simulink model "Comprobar_Posicion_PID_ISA"  (R2021b)
settings: Solver=ode45  StartTime=0.0  StopTime=100  RelTol=1e-3  EnableMultiTasking=on
undefined symbols (not defined in the file or in its folder): airspeed_0, alpha_0, altitude_0, beta_0, deflect_sat, Earth, euler_0, h0, JSBSim, local_V_0, mTotal, Pos_0, pqr_0, r_MotorLeft, r_MotorRight, theta_0, Vel_0, VTOL_FW, WGS84
libraries: simulink_need_slupdate x5, aerolibfltsims x4, sharedutil x3, sharedtransform x2, aerolibtransform2 x1, aerolibutil x1
(part 2 of 2)

== matlab function Comprobar_Posicion_PID_ISA/Control de Actitud/Dynamic Model/VSkye/Ecuaciones_de_Navegacion1 ==
  data: Mm output; input input
function Mm=par_Motor(input)
%g=9.81;
C_P=0.04;
C_T=0.08;
INCH2M=2.54e-2;
D=8*INCH2M;
Kpar=-D*C_P/(2*pi()*C_T);
%Ft=(1/3.27193530612245)*(-0.0292*(input*100).^2 + 36.681*(input*100) - 107.5)*g/1000;%en N;
Ft=-9.8*input;
Par=Kpar*Ft;%en Nm;

Mm=[0;0;Par];
end

== matlab function Comprobar_Posicion_PID_ISA/Control de Actitud/Lamda controller/PID ISA1/PID CPOH ==
  data: sp input; vm output; vc input; Kc input; Ti input; Td input; Ts input; u0 input; Min_U input; Max_U input; ui1 input; ekf1 input; ui output; ekf output
function [vm,ui,ekf] = fcn(sp,vc,Kc,Ti,Td,Ts,u0,Min_U,Max_U,ui1,ekf1)

% Variables auxiliares...
N =0;         % N=0 desconecta el filtro de la derivada
b  = 1;       % Ponderación de la ref en la acción Proporcional
c  = 1;       % Ponderación de la ref en la acción derivada
offset = u0;  % offset, incluye el efecto de los puntos de
ki = 0;

if (Ti~=0)
    ki = (Kc*Ts)/Ti;
end

kd = (Kc*Td)/Ts;

if N~=0
    kn =Td/(N*Ts);
end

tauf = 0;
kf = tauf/Ts;

% Filtrado de la medida
if tauf == 0
    ykf=vc;
else
    ykf=(kf*ykf1+vc)/(kf+1);
end

% cálculo termino proporcional...
% con ponderacion de la referencia...
up=Kc*(b*sp-ykf);

% cálculo del termino derivada...
% con ponderacion de la referencia...
% y filtrado...

if (Td==0)
    ud=0;
    ekf=0;
else
    ek=c*sp-ykf;
    if N==0
        ekf=ek;
    else
        ekf=(kn*ekf1+ek)/(kn+1);
    end
    ud=kd*(ekf-ekf1);
end

% cálculo termino integral...
if (Ti==0)
    ui=0;
else
    ui=ui1+ki*(sp-ykf);
end
vm = up+ui+ud+offset;

% Antiwindup...
% saturación del incremento mínimo (El incremento mínimo es de 0.005 mm)
% saturación de la acción de control.
if (vm < Min_U)
    ui=ui1;
    vm=Min_U;
end
if (vm > Max_U)
    ui=ui1;
    vm= Max_U;
end

== matlab function Comprobar_Posicion_PID_ISA/Control de Actitud/Dynamic Model/VSkye/Ecuaciones_de_Navegacion ==
  data: xe_dot output; euler input; ye_dot output; ze_dot output; Vels input
function [xe_dot,ye_dot,ze_dot] = fcn(euler,Vels)

roll=euler(1);
pitch=euler(2);
yaw=euler(3);

Cx=[[1 0 0];[0 cos(roll) sin(roll)];[0 -sin(roll) cos(roll)]];
Cy=[[cos(pitch) 0 -sin(pitch)];[0 1 0];[sin(pitch) 0 cos(pitch)]];
Cz=[[cos(yaw) sin(yaw) 0];[-sin(yaw) cos(yaw) 0];[0 0 1]];

NAV_vect=((Cx*Cy*Cz)')*[Vels(1);Vels(2);Vels(3)];

xe_dot=NAV_vect(1);
ye_dot=NAV_vect(2);
ze_dot=NAV_vect(3);
end

% function [xe_dot,ye_dot,he_dot] = fcn(euler,Vels)
% V=sqrt(Vels(1)^2+Vels(2)^2+Vels(3)^2);
% alpha = atan2(Vels(3),Vels(1));
% beta  = asin(Vels(2)/V);
% 
% xe_dot=V*cos(alpha)*cos(beta)*cos(euler(3))*cos(euler(2)) + V*sin(beta)*(cos(euler(3)*sin(euler(2))*sin(euler(1)) - sin(euler(3))*cos(euler(1)))) + V*sin(alpha)*cos(beta)*(cos(euler(3))*sin(euler(2))*cos(euler(1)) + sin(euler(3))*sin(euler(1)));
% ye_dot=V*cos(alpha)*cos(beta)*sin(euler(3))*cos(euler(2)) + V*sin(beta)*(sin(euler(3))*sin(euler(2))*sin(euler(1)) - cos(euler(3))*cos(euler(1))) + V*sin(alpha)*cos(beta)*(sin(euler(3))*sin(euler(2))*sin(euler(1)) - cos(euler(3))*sin(euler(1)));
% he_dot=V*cos(alpha)*cos(beta)*sin(euler(2)) - V*sin(beta)*cos(euler(2))*sin(euler(1)) - V*sin(alpha)*cos(beta)*cos(euler(2))*cos(euler(1));
% 
% end
